simulink model "ModelMultirate"  (R2014a)
settings: Solver=ode3  StartTime=0.0  StopTime=20  FixedStep=0.01  RelTol=1e-3
settings Model: Creator=lgw  LastModifiedBy=李广文

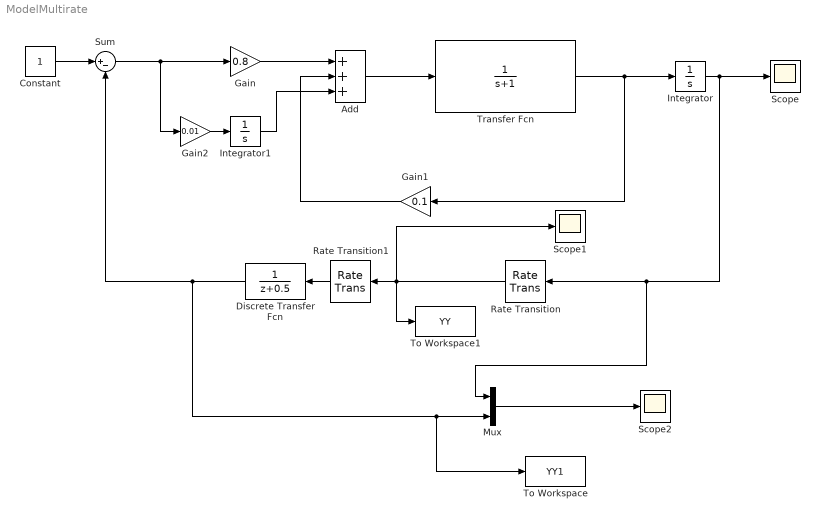
== system ModelMultirate ==
  Add : Sum  Inputs=+++
  Constant : Constant
  Discrete Transfer Fcn : DiscreteTransferFcn  SampleTime=0.01
  Gain : Gain  Gain=0.8
  Gain1 : Gain  Gain=0.1
  Gain2 : Gain  Gain=0.01
  Integrator : Integrator
  Integrator1 : Integrator
  Mux : Mux  Inputs=2
  Rate Transition : RateTransition  OutPortSampleTime=0.05
  Rate Transition1 : RateTransition  OutPortSampleTime=0.01
  Scope : Scope
  Scope1 : Scope
  Scope2 : Scope
      settings: SaveName=ScopeData2
  Sum : Sum  Inputs=|+-
  To Workspace : ToWorkspace  VariableName=YY1  SampleTime=-1
  To Workspace1 : ToWorkspace  VariableName=YY  SampleTime=-1
  Transfer Fcn : TransferFcn  Denominator=[1 1]
  wires:
  Transfer Fcn/1 -> Gain1/1, Integrator/1
  Integrator/1 -> Scope/1, Rate Transition/1, Mux/1
  Constant/1 -> Sum/1
  Add/1 -> Transfer Fcn/1
  Sum/1 -> Gain2/1, Gain/1
  Gain/1 -> Add/1
  Gain1/1 -> Add/2
  Integrator1/1 -> Add/3
  Gain2/1 -> Integrator1/1
  Mux/1 -> Scope2/1
  Discrete Transfer Fcn/1 -> To Workspace/1, Mux/2, Sum/2
  Rate Transition/1 -> Rate Transition1/1, Scope1/1, To Workspace1/1
  Rate Transition1/1 -> Discrete Transfer Fcn/1
